simulink model "Lab1_parameter_estimation_student"  (R2024b)
settings: Solver=FixedStepAuto  StartTime=0.0  StopTime=30  FixedStep=0.001  RelTol=1e-3
values from neighbouring files (symbols this model uses):
  motor_B = 0.0001    [Lab1_motor_params_student.m]
  motor_Eff = 0.5    [Lab1_motor_params_student.m]
  motor_J = 0.001    [Lab1_motor_params_student.m]
  motor_Ke = 0.05    [Lab1_motor_params_student.m]
  motor_L = 0.00284    [Lab1_motor_params_student.m]
  motor_R = 3.18    [Lab1_motor_params_student.m]
libraries: simulink x2
settings Model: Creator=tanawatp  LastModifiedBy=pboon
settings DataIOCC: OutputOption=AdditionalOutputTimes  OutputTimes=SDO_OutputTimes  ReturnWorkspaceOutputsName=SDOSimTest_Log
settings RTWCC: GPUComputeCapability=3.5

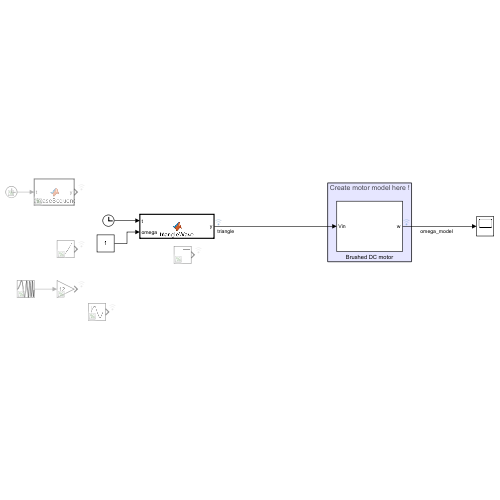
[thumbnail: Simulink's stored preview of the top-level diagram]
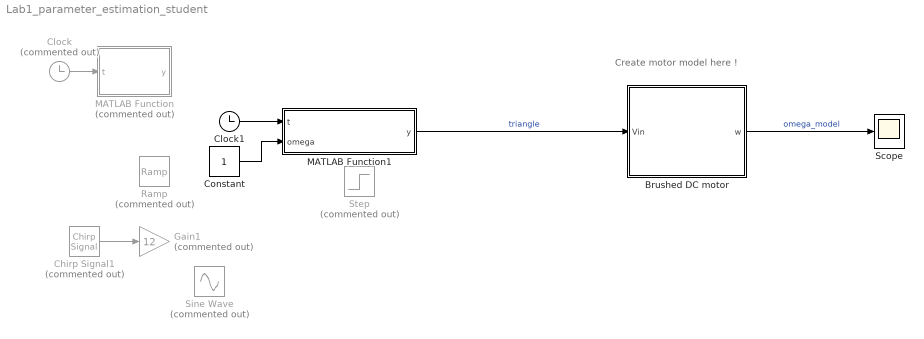
== system Lab1_parameter_estimation_student ==
  note: Create motor model here !
  Brushed DC motor : Subsystem
  Chirp Signal1 : simulink/Sources/Chirp Signal  Commented=on  f1=0  T=30  f2=2
  Clock : Clock  Commented=on
  Clock1 : Clock
  Constant : Constant
  Gain1 : Gain  Commented=on  Gain=12
  MATLAB Function : MATLAB Function  Commented=on  TreatAsAtomicUnit=on
  MATLAB Function1 : MATLAB Function  TreatAsAtomicUnit=on
  Ramp : simulink/Sources/Ramp  Commented=on  slope=0.4  start=0  InitialOutput=0
  Scope : Scope
  Sine Wave : Sin  Commented=on  Amplitude=12  Frequency=1/4  SampleTime=0
  Step : Step  Commented=on  Time=4  After=12  SampleTime=0
  wires:
  Brushed DC motor/1(w) -> Scope/1  "omega_model"
  Clock1/1 -> MATLAB Function1/1(t)
  Constant/1 -> MATLAB Function1/2(omega)
  Chirp Signal1/1 -> Gain1/1
  Clock/1 -> MATLAB Function/1(t)
  MATLAB Function1/1(y) -> Brushed DC motor/1(Vin)  "triangle"

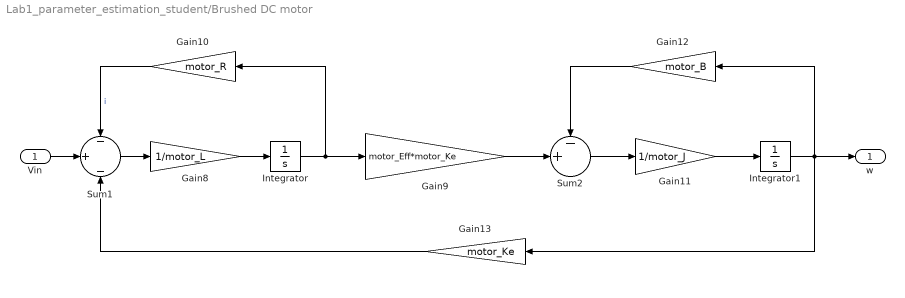
== system Lab1_parameter_estimation_student/Brushed DC motor ==
  Vin : Inport
  Gain10 : Gain  Gain=motor_R
  Gain11 : Gain  Gain=1/motor_J
  Gain12 : Gain  Gain=motor_B
  Gain13 : Gain  Gain=motor_Ke
  Gain8 : Gain  Gain=1/motor_L
  Gain9 : Gain  Gain=motor_Eff*motor_Ke
  Integrator : Integrator
  Integrator1 : Integrator
  Sum1 : Sum  Inputs=-|+|-
  Sum2 : Sum  Inputs=-+|
  w : Outport
  wires:
  Gain8/1 -> Integrator/1
  Integrator/1 -> Gain9/1, Gain10/1
  Vin/1 -> Sum1/2
  Sum1/1 -> Gain8/1
  Gain10/1 -> Sum1/1  "i"
  Gain9/1 -> Sum2/2
  Sum2/1 -> Gain11/1
  Gain11/1 -> Integrator1/1
  Gain12/1 -> Sum2/1
  Integrator1/1 -> Gain13/1, w/1, Gain12/1
  Gain13/1 -> Sum1/3

== matlab function Lab1_parameter_estimation_student/MATLAB Function ==
  data: t input; y output
function y = staircaseSequence(t)
%#codegen
% This function outputs a sequence with an "on" time of 3 seconds and an "off"
% time of 2 seconds. The "on" time corresponds to outputting the next number
% in the sequence, and the "off" time corresponds to outputting 0.

% Define the sequence vector.
seq = [0, 3, 4, 5, 6, 7, 8, 9, 10, 11, 12];

% Total number of elements in the sequence.
N = length(seq);

% Define the on and off times.
onTime = 3;  % 3 seconds for on time
offTime = 2; % 2 seconds for off time

% Compute the total cycle time (on time + off time).
cycleTime = onTime + offTime;

% Determine the current cycle index based on the simulation time.
cycleIndex = mod(t, cycleTime);

% Calculate the sequence index.
seqIndex = floor(t / cycleTime) + 1;

% Wrap the sequence index to repeat the sequence.
seqIndex = mod(seqIndex-1, N) + 1;

% Output the value based on whether we are in the "on" or "off" period.
if cycleIndex < onTime
    % During "on" time, output the sequence value.
    y = seq(seqIndex);
else
    % During "off" time, output 0.
    y = 0;
end

== matlab function Lab1_parameter_estimation_student/MATLAB Function1 ==
  data: t input; y output; omega input
function y = triangleWave(t, omega)
%#codegen
% This function outputs a unipolar triangle wave that:
%   - Starts at 0 at time t = 0,
%   - Rises linearly to 12 at t = T/2,
%   - Then falls linearly back to 0 at t = T.
%
% The waveform repeats every T = 2*pi/omega seconds.
%
% Inputs:
%   t     - time value (scalar)
%   omega - angular frequency in rad/s (e.g., 1, 1/4, or 4)

% Compute the period based on the desired angular frequency.
T = 2*pi/omega;   % period corresponding to angular frequency omega
A = 12;           % peak value of the triangle wave

% Compute the time within the current period.
t_mod = mod(t, T);

% Compute the triangle wave value.
if t_mod < T/2  
    % Rising portion: y increases linearly from 0 to 12.
    y = (A/(T/2)) * t_mod;
else           
    % Falling portion: y decreases linearly from 12 back to 0.
    y = A - (A/(T/2)) * (t_mod - T/2);
end
